simulink model "heli_sim"  (R2014a)
settings: Solver=ode45  StartTime=0.0  StopTime=10  RelTol=1e-3
values from neighbouring files (symbols this model uses):
  heli_sys = sys_class    [create_all_sys.m]
  sysr = ss(A_r,B_r,C_r,0)    [model_reduction.m]
undefined symbols (not defined in the file or in its folder): sysb, sysb_x0, sysr_x0
settings Model: Creator=UX31  LastModifiedBy=UX31

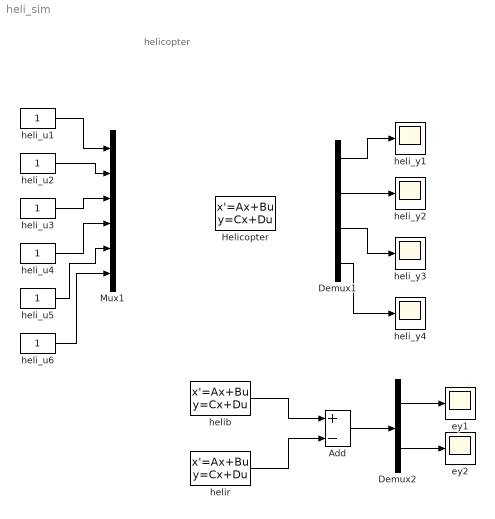
== system heli_sim ==
  note: helicopter
  Add : Sum  Inputs=+-
  Demux1 : Demux
  Demux2 : Demux  Outputs=2
  Helicopter : StateSpace  A=heli_sys.sys.a  B=heli_sys.sys.b  C=heli_sys.sys.c  D=heli_sys.sys.d  X0=heli_sys.x0_lb
  Mux1 : Mux  Inputs=6
  ey1 : Scope
  ey2 : Scope
  heli_u{1..6} (6 alike) : Constant
  heli_y{1..4} (4 alike) : Scope
      heli_y1 settings: SaveName=ScopeData8
      heli_y2 settings: SaveName=ScopeData9
      heli_y3 settings: SaveName=ScopeData10
      heli_y4 settings: SaveName=ScopeData11
  helib : StateSpace  A=sysb.sys.a  B=sysb.sys.b  C=sysb.sys.c  D=sysb.sys.d  X0=sysb_x0
  helir : StateSpace  A=sysr.sys.a  B=sysr.sys.b  C=sysr.sys.c  D=sysr.sys.d  X0=sysr_x0
  wires:
  heli_u1/1 -> Mux1/1
  heli_u2/1 -> Mux1/2
  heli_u3/1 -> Mux1/3
  heli_u4/1 -> Mux1/4
  heli_u5/1 -> Mux1/5
  heli_u6/1 -> Mux1/6
  Demux1/1 -> heli_y1/1
  Demux1/2 -> heli_y2/1
  Demux1/3 -> heli_y3/1
  Demux1/4 -> heli_y4/1
  helib/1 -> Add/1
  helir/1 -> Add/2
  Add/1 -> Demux2/1
  Demux2/2 -> ey2/1
  Demux2/1 -> ey1/1
